simulink model "ex00_model"  (R2023a)
settings: Solver=FixedStepDiscrete  StartTime=0.0  StopTime=T_s*length(x_0)  RelTol=1e-3
values from neighbouring files (symbols this model uses):
  T_s = 1/F_s    (= 6.25e-05)    [ex00_config.m]
undefined symbols (not defined in the file or in its folder): fir_num, iir_den, iir_num
libraries: dspsrcs4 x2
settings Model: Creator=daniele  LastModifiedBy=daniele

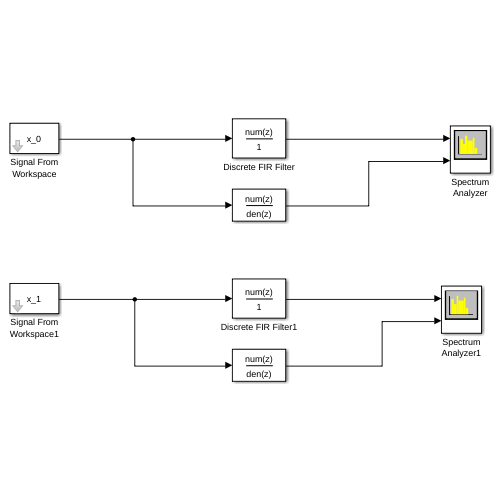
[thumbnail: Simulink's stored preview of the top-level diagram]
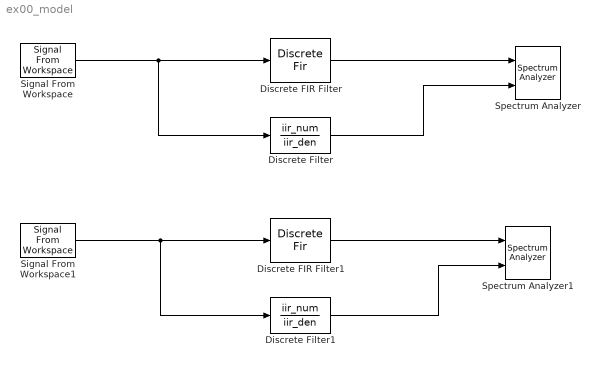
== system ex00_model ==
  Discrete FIR Filter : DiscreteFir  Coefficients=fir_num
  Discrete FIR Filter1 : DiscreteFir  Coefficients=fir_num
  Discrete Filter : DiscreteFilter  Numerator=iir_num  Denominator=iir_den
  Discrete Filter1 : DiscreteFilter  Numerator=iir_num  Denominator=iir_den
  Signal From Workspace : dspsrcs4/Signal From Workspace  X=x_0  Ts=T_s  nsamps=1  OutputAfterFinalValue=Setting to zero  ignoreOrWarnInputAndFrameLengths=off  OutputFrames=off
  Signal From Workspace1 : dspsrcs4/Signal From Workspace  X=x_1  Ts=T_s  nsamps=1  OutputAfterFinalValue=Setting to zero  ignoreOrWarnInputAndFrameLengths=off  OutputFrames=off
  Spectrum Analyzer : SpectrumAnalyzer  NumInputPorts=2  YLimits=[-20 80]  ColorLimits=[-20 80]  DefaultConfigurationName=spbscopes.SpectrumAnalyzerBlockCfg  IsFrequencyInputMode=0  FrequencyVectorPort=0  FrequencyVectorFromPort=0  FrequencyInputRBWPort=0  FrequencyInputRBWFromPort=0
  Spectrum Analyzer1 : SpectrumAnalyzer  NumInputPorts=2  YLimits=[-20 80]  ColorLimits=[-20 80]  DefaultConfigurationName=spbscopes.SpectrumAnalyzerBlockCfg  IsFrequencyInputMode=0  FrequencyVectorPort=0  FrequencyVectorFromPort=0  FrequencyInputRBWPort=0  FrequencyInputRBWFromPort=0
  wires:
  Signal From Workspace1/1 -> Discrete Filter1/1, Discrete FIR Filter1/1
  Signal From Workspace/1 -> Discrete Filter/1, Discrete FIR Filter/1
  Discrete FIR Filter/1 -> Spectrum Analyzer/1
  Discrete Filter/1 -> Spectrum Analyzer/2
  Discrete FIR Filter1/1 -> Spectrum Analyzer1/1
  Discrete Filter1/1 -> Spectrum Analyzer1/2
